simulink model "CSI_0313_4DC"  (R2018a)
settings: Solver=FixedStepDiscrete  StartTime=0.0  StopTime=Tstop  FixedStep=Tdelt  MaxStep=1e-4  RelTol=1e-3
values from neighbouring files (symbols this model uses):
  C = 12e-6    (= 1.2e-05)    [Inputparameter.m]
  Cdc = 4.76*10^-3    (= 0.00476)    [Inputparameter.m]
  Cemc = 1.5e-6    (= 1.5e-06)    [Inputparameter.m]
  fanalog = 7000    [Run.m]
  fKIUdc = 6    [Run.m]
  fKPUdc = 0.4    [Run.m]
  fTs = Update/18000    (= 0.000111111111111)    [Run.m]
  K120 = 0.0    (= 0)    [Run.m]
  K21 = 0.0    (= 0)    [Run.m]
  K5 = 0.0    (= 0)    [Run.m]
  K7 = 0.0    (= 0)    [Run.m]
  Kipll = 1.0    (= 1)    [Run.m]
  klmt = 0.3    [Run.m]
  Kpll = 20.0    (= 20)    [Run.m]
  Lgrid = 7.717e-4*10    (= 0.007717)    [Run.m]
  Lline = 60e-6    (= 6e-05)    [Inputparameter.m]
  Lpwm = 184.8e-6    (= 0.0001848)    [Inputparameter.m]
  mode = 1    [Run.m]
  Nsw = 18000/fbase    [Run.m]
  Qbpf = 1.0    (= 1)    [Run.m]
  Rc = 10e-3    (= 0.01)    [Inputparameter.m]
  Remc = 1e-3    (= 0.001)    [Inputparameter.m]
  Rgrid = 2*pi*fbase*Lgrid/XR    [Run.m]
  Rline = 4.95e-3    (= 0.00495)    [Inputparameter.m]
  Rpre = 2.2    [Inputparameter.m]
  Rpwm = 6.2e-3    (= 0.0062)    [Inputparameter.m]
  Tdelt = (fTs)/(200*Update)    (= 2.77777777778e-07)    [Run.m]
  Tdt = 1.27e-6    (= 1.27e-06)    [Run.m]
  tstart = 0.2    [Run.m]
  Tvstep = 1.5    [Run.m]
  Update = 2    [Run.m]
  Vbase = 400*sqrt(2/3)    [Inputparameter.m]
undefined symbols (not defined in the file or in its folder): sigbuilder_block
libraries: powerlib x412
(part 2 of 13)

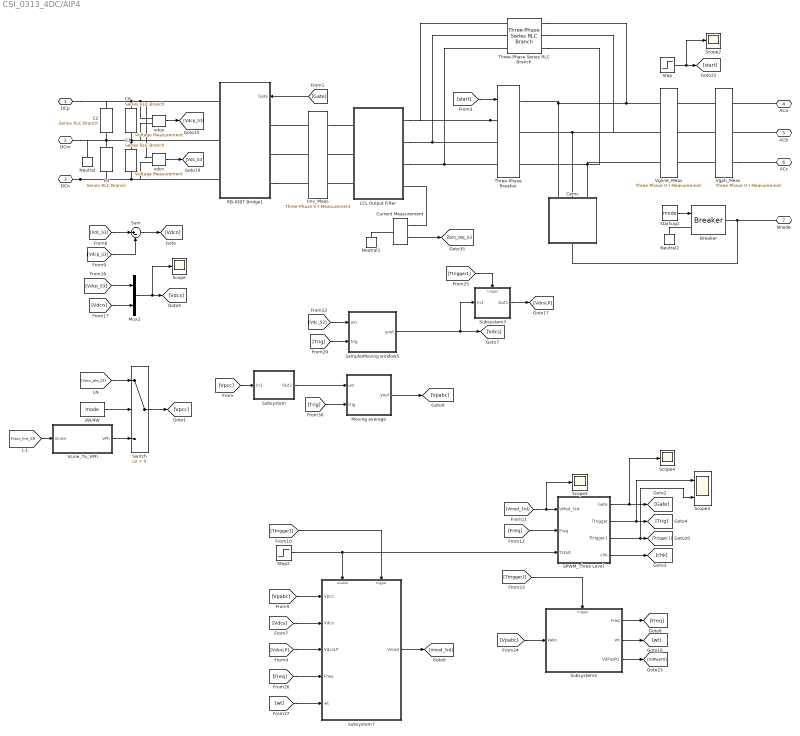
== system CSI_0313_4DC/AIP4 ==
  3W/4W : Constant  Value=mode
  Breaker : powerlib/Elements/Breaker  InitialState=0  SwitchingTimes="[1/60  5/60]"  External=on  BreakerResistance=1e-6  SnubberResistance=1e6  SnubberCapacitance=inf  Measurements=None  MoreParameters=on  NoBreakLoop=off
      settings: SourceProductName=Simscape Electrical
  C1 : powerlib/Elements/Series RLC Branch  LConnTagsString=__new0  RConnTagsString=__new0  BranchType=C  Resistance=Rc  Inductance=Lpwm  SetiL0=off  InitialCurrent=0  Capacitance=Cdc  Setx0=on  InitialVoltage=320  Measurements=None
      settings: SourceProductName=Simscape Electrical
  C2 : powerlib/Elements/Series RLC Branch  LConnTagsString=__new0  RConnTagsString=__new0  BranchType=R  Resistance=120e3  Inductance=Lpwm  SetiL0=off  InitialCurrent=0  Capacitance=Cdc  Setx0=on  InitialVoltage=300  Measurements=None
      settings: SourceProductName=Simscape Electrical
  C3 : powerlib/Elements/Series RLC Branch  LConnTagsString=__new0  RConnTagsString=__new0  BranchType=R  Resistance=120e3  Inductance=Lpwm  SetiL0=off  InitialCurrent=0  Capacitance=Cdc  Setx0=on  InitialVoltage=300  Measurements=None
      settings: SourceProductName=Simscape Electrical
  C8 : powerlib/Elements/Series RLC Branch  LConnTagsString=__new0  RConnTagsString=__new0  BranchType=C  Resistance=Rc  Inductance=Lpwm  SetiL0=off  InitialCurrent=0  Capacitance=Cdc  Setx0=on  InitialVoltage=320  Measurements=None
      settings: SourceProductName=Simscape Electrical
  Cemc : Subsystem
  Current Measurement : powerlib/Measurements/Current Measurement  PhasorSimulation=off  OutputType=Complex  PSBequivalent=0
      settings: SourceProductName=Simscape Electrical
  Iinv_Meas : powerlib/Measurements/Three-Phase V-I Measurement  VoltageMeasurement=no  SetLabelV=off  LabelV=Vabc  Vpu=off  VpuLL=off  CurrentMeasurement=yes  SetLabelI=on  LabelI=Iinv_S3  Ipu=off  Pbase=100e6  Vbase=500e3  OutputType=Complex  PhasorSimulation=off  PSBequivalent=0
      settings: SourceProductName=Simscape Electrical
  LCL Output Filter : Subsystem  AncestorBlock=AIP_Library0107/LCL Output Filter
  Moving average : MATLAB Function  Priority=-1  AncestorBlock=AIP_Library0123/Sample//Moving window  TreatAsAtomicUnit=on  mask{iNumAvg=4, iNumDly=1, ubase=1}
      mask prompts: iNumAvg "Sample points"; iNumDly "Delay points"; ubase "Base Value"
  Mux2 : Mux  Inputs=2
  Neutral : powerlib/Elements/Neutral  LConnTagsString=a  NodeNumber=10
      settings: SourceProductName=Simscape Electrical  SourceProductBaseCode=PS
  Neutral1 : powerlib/Elements/Neutral  LConnTagsString=a  NodeNumber=10
      settings: SourceProductName=Simscape Electrical  SourceProductBaseCode=PS
  Neutral2 : powerlib/Elements/Neutral  LConnTagsString=a  NodeNumber=10
      settings: SourceProductName=Simscape Electrical  SourceProductBaseCode=PS
  RB-IGBT Bridge1 : Subsystem  AncestorBlock=AIP_Library0107/RB-IGBT Bridge
  SPWM_Three Level : Subsystem  mask{ID=1, Tdelt=Tdelt, Tdt=Tdt}
      mask prompts: ID "Unit Serial Number"; Tdelt "Simulation Step [s]"; Tdt "Dead time [s]"
  Sample/Moving window5 : MATLAB Function  Priority=-1  AncestorBlock=AIP_Library0123/Sample//Moving window  TreatAsAtomicUnit=on  mask{iNumAvg=1, iNumDly=1, ubase=1}
      mask prompts: iNumAvg "Sample points"; iNumDly "Delay points"; ubase "Base Value"
  Scope{,2,4..5} (4 alike) : Scope
  Scope3 : Scope  NumInputPorts=2
  Startsig1 : Constant  Value=mode
  Step : Step  Time=0.25  SampleTime=0
  Step2 : Step  Time=0.25  SampleTime=0
  Subsystem : Subsystem
  Subsystem3 : Subsystem
  Subsystem5 : Subsystem
  Subsystem7 : Subsystem
  Sum : Sum  Inputs=|+-
  Switch : Switch  Criteria=u2 > Threshold
  Three-Phase Series RLC Branch : powerlib/Elements/Three-Phase Series RLC Branch  LConnTagsString=A|B|C  RConnTagsString=A|B|C  BranchType=R  Resistance=Rpre  Inductance=1e-3  Capacitance=1e-6  Measurements=None
      settings: SourceProductName=Simscape Electrical
  Three-Phase Breaker : powerlib/Elements/Three-Phase Breaker  InitialState=open  SwitchA=on  SwitchB=on  SwitchC=on  SwitchTimes=tstart  External=on  BreakerResistance=1e-6  SnubberResistance=1e6  SnubberCapacitance=inf  Measurements=None
      settings: SourceProductName=Simscape Electrical
  VLine_To_VPh : MATLAB Function  AncestorBlock=AIP_Library0107/VLine_To_VPh  TreatAsAtomicUnit=on
  Vgline_Meas : powerlib/Measurements/Three-Phase V-I Measurement  VoltageMeasurement=phase-to-phase  SetLabelV=on  LabelV=Vpcc_line_S3  Vpu=off  VpuLL=off  CurrentMeasurement=no  SetLabelI=off  LabelI=vpccabbc  Ipu=off  Pbase=100e6  Vbase=500e3  OutputType=Complex  PhasorSimulation=off  PSBequivalent=0
      settings: SourceProductName=Simscape Electrical
  Vgph_Meas : powerlib/Measurements/Three-Phase V-I Measurement  VoltageMeasurement=phase-to-ground  SetLabelV=on  LabelV=Vpcc_phn_S3  Vpu=off  VpuLL=off  CurrentMeasurement=no  SetLabelI=off  LabelI=vpccabbc  Ipu=off  Pbase=100e6  Vbase=500e3  OutputType=Complex  PhasorSimulation=off  PSBequivalent=0
      settings: SourceProductName=Simscape Electrical
  vdcn : powerlib/Measurements/Voltage Measurement  PhasorSimulation=off  OutputType=Magnitude  PSBequivalent=0
      settings: SourceProductName=Simscape Electrical
  vdcp : powerlib/Measurements/Voltage Measurement  PhasorSimulation=off  OutputType=Magnitude  PSBequivalent=0
      settings: SourceProductName=Simscape Electrical
  DCp : PMIOPort  Side=Left
  DCm : PMIOPort  Port=2  Side=Left
  DCn : PMIOPort  Port=3  Side=Left
  ACa : PMIOPort  Port=4  Side=Right
  ACb : PMIOPort  Port=5  Side=Right
  ACc : PMIOPort  Port=6  Side=Right
  Nnode : PMIOPort  Port=7  Side=Right
  tag scope: Zero_seq_S3=global
  wires:
  [wt] -> Subsystem7/5(wt)
  Subsystem5/3(VdPosPU) -> [VdPosPU]
  Subsystem5/2(wt) -> [wt]
  [Freq] -> Subsystem7/4("Freq ")
  [Vpabc] -> Subsystem5/1(Vabc)
  [Ttrigger1] -> Subsystem5/Trigger
  Sample/Moving window5/1(yout) -> [Vdcs], Subsystem3/1(In1)
  [Vdc_S3] -> Sample/Moving window5/1(uin)
  Sum/1 -> [Vdcn]
  [Vdcp_S3] -> Sum/2
  [Vdc_S3] -> Sum/1
  [VdcsLP] -> Subsystem7/3(VdcsLP)
  Subsystem3/1(Out1) -> [VdcsLP]
  Step2/1 -> Subsystem7/Enable, SPWM_Three Level/3(Tstart)
  [start] -> Three-Phase Breaker/1
  [Ttrigger1] -> Subsystem3/Trigger
  [Trig] -> Sample/Moving window5/2(trig)
  vdcp/1 -> [Vdcp_S3]
  Startsig1/1 -> Breaker/1
  Step/1 -> [start], Scope2/1
  [Gate] -> RB-IGBT Bridge1/1(Gate)
  vdcn/1 -> [Vdc_S3]
  Current Measurement/1 -> [Zero_seq_S3]
  [Freq] -> SPWM_Three Level/2(Freq)
  [Vmod_3rd] -> Scope5/1, SPWM_Three Level/1(VMod_3rd)
  Subsystem5/1(Freq) -> [Freq]
  Subsystem7/1(Vmod) -> [Vmod_3rd]
  [Ttrigger1] -> Subsystem7/Trigger
  [Vdcs] -> Subsystem7/2(Vdcs)
  [Vpabc] -> Subsystem7/1(Vpcc)
  [Vdcn] -> Mux2/2
  [Vdcp_S3] -> Mux2/1
  SPWM_Three Level/4(chk) -> [chk]
  SPWM_Three Level/3(Ttrigger1) -> [Ttrigger1], Scope3/2
  SPWM_Three Level/1(Gate) -> [Gate], Scope4/1
  Mux2/1 -> [Vdcx], Scope/1
  SPWM_Three Level/2(Ttrigger) -> [Trig], Scope3/1
  Switch/1 -> [Vpcc]
  [Vpcc_phn_S3] -> Switch/1
  Subsystem/1(Out1) -> Moving average/1(uin)
  [Trig] -> Moving average/2(trig)
  Moving average/1(yout) -> [Vpabc]
  VLine_To_VPh/1(VPh) -> Switch/3
  [Vpcc_line_S3] -> VLine_To_VPh/1(VLine)
  [Vpcc] -> Subsystem/1(In1)
  3W/4W/1 -> Switch/2
  connections:
  Current Measurement/RConn1 -- LCL Output Filter/RConn4
  LCL Output Filter/LConn3 -- Iinv_Meas/RConn3
  Vgph_Meas/LConn3 -- Vgline_Meas/RConn3
  Vgph_Meas/LConn1 -- Vgline_Meas/RConn1
  LCL Output Filter/LConn2 -- Iinv_Meas/RConn2
  Iinv_Meas/RConn1 -- LCL Output Filter/LConn1
  RB-IGBT Bridge1/LConn1 -- Iinv_Meas/LConn1
  ACb/RConn1 -- Vgph_Meas/RConn2
  Vgph_Meas/LConn2 -- Vgline_Meas/RConn2
  Vgph_Meas/RConn3 -- ACc/RConn1
  RB-IGBT Bridge1/LConn3 -- Iinv_Meas/LConn3
  Neutral2/LConn1 -- Breaker/LConn1
  RB-IGBT Bridge1/LConn2 -- Iinv_Meas/LConn2
  ACa/RConn1 -- Vgph_Meas/RConn1
  Current Measurement/LConn1 -- Neutral1/LConn1
  Three-Phase Breaker/LConn1 -- LCL Output Filter/RConn1 -- Three-Phase Series RLC Branch/LConn1
  DCn/RConn1 -- C3/RConn1 -- C1/RConn1 -- vdcn/LConn2 -- RB-IGBT Bridge1/RConn3
  Nnode/RConn1 -- Breaker/RConn1 -- Cemc/RConn1
  Three-Phase Series RLC Branch/LConn2 -- LCL Output Filter/RConn2 -- Three-Phase Breaker/LConn2
  Cemc/LConn2 -- Three-Phase Series RLC Branch/RConn2 -- Vgline_Meas/LConn2 -- Three-Phase Breaker/RConn2
  Three-Phase Series RLC Branch/LConn3 -- LCL Output Filter/RConn3 -- Three-Phase Breaker/LConn3
  C1/LConn1 -- vdcp/LConn2 -- RB-IGBT Bridge1/RConn2 -- C2/RConn1 -- Neutral/LConn1 -- DCm/RConn1 -- C3/LConn1 -- C8/RConn1
  Cemc/LConn3 -- Three-Phase Series RLC Branch/RConn3 -- Vgline_Meas/LConn3 -- Three-Phase Breaker/RConn3
  Cemc/LConn1 -- Three-Phase Breaker/RConn1 -- Three-Phase Series RLC Branch/RConn1 -- Vgline_Meas/LConn1
  C8/LConn1 -- DCp/RConn1 -- C2/LConn1 -- RB-IGBT Bridge1/RConn1 -- vdcn/LConn1 -- vdcp/LConn1

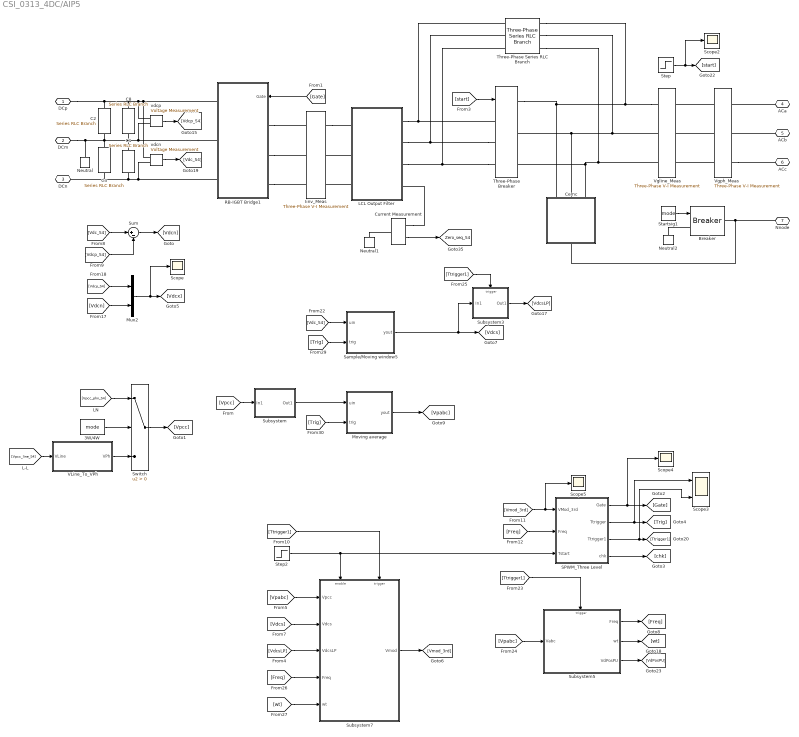
== system CSI_0313_4DC/AIP5 ==
  3W/4W : Constant  Value=mode
  Breaker : powerlib/Elements/Breaker  InitialState=0  SwitchingTimes="[1/60  5/60]"  External=on  BreakerResistance=1e-6  SnubberResistance=1e6  SnubberCapacitance=inf  Measurements=None  MoreParameters=on  NoBreakLoop=off
      settings: SourceProductName=Simscape Electrical
  C1 : powerlib/Elements/Series RLC Branch  LConnTagsString=__new0  RConnTagsString=__new0  BranchType=C  Resistance=Rc  Inductance=Lpwm  SetiL0=off  InitialCurrent=0  Capacitance=Cdc  Setx0=on  InitialVoltage=320  Measurements=None
      settings: SourceProductName=Simscape Electrical
  C2 : powerlib/Elements/Series RLC Branch  LConnTagsString=__new0  RConnTagsString=__new0  BranchType=R  Resistance=120e3  Inductance=Lpwm  SetiL0=off  InitialCurrent=0  Capacitance=Cdc  Setx0=on  InitialVoltage=300  Measurements=None
      settings: SourceProductName=Simscape Electrical
  C3 : powerlib/Elements/Series RLC Branch  LConnTagsString=__new0  RConnTagsString=__new0  BranchType=R  Resistance=120e3  Inductance=Lpwm  SetiL0=off  InitialCurrent=0  Capacitance=Cdc  Setx0=on  InitialVoltage=300  Measurements=None
      settings: SourceProductName=Simscape Electrical
  C8 : powerlib/Elements/Series RLC Branch  LConnTagsString=__new0  RConnTagsString=__new0  BranchType=C  Resistance=Rc  Inductance=Lpwm  SetiL0=off  InitialCurrent=0  Capacitance=Cdc  Setx0=on  InitialVoltage=320  Measurements=None
      settings: SourceProductName=Simscape Electrical
  Cemc : Subsystem
  Current Measurement : powerlib/Measurements/Current Measurement  PhasorSimulation=off  OutputType=Complex  PSBequivalent=0
      settings: SourceProductName=Simscape Electrical
  Iinv_Meas : powerlib/Measurements/Three-Phase V-I Measurement  VoltageMeasurement=no  SetLabelV=off  LabelV=Vabc  Vpu=off  VpuLL=off  CurrentMeasurement=yes  SetLabelI=on  LabelI=Iinv_S4  Ipu=off  Pbase=100e6  Vbase=500e3  OutputType=Complex  PhasorSimulation=off  PSBequivalent=0
      settings: SourceProductName=Simscape Electrical
  LCL Output Filter : Subsystem  AncestorBlock=AIP_Library0107/LCL Output Filter
  Moving average : MATLAB Function  Priority=-1  AncestorBlock=AIP_Library0123/Sample//Moving window  TreatAsAtomicUnit=on  mask{iNumAvg=4, iNumDly=1, ubase=1}
      mask prompts: iNumAvg "Sample points"; iNumDly "Delay points"; ubase "Base Value"
  Mux2 : Mux  Inputs=2
  Neutral : powerlib/Elements/Neutral  LConnTagsString=a  NodeNumber=10
      settings: SourceProductName=Simscape Electrical  SourceProductBaseCode=PS
  Neutral1 : powerlib/Elements/Neutral  LConnTagsString=a  NodeNumber=10
      settings: SourceProductName=Simscape Electrical  SourceProductBaseCode=PS
  Neutral2 : powerlib/Elements/Neutral  LConnTagsString=a  NodeNumber=10
      settings: SourceProductName=Simscape Electrical  SourceProductBaseCode=PS
  RB-IGBT Bridge1 : Subsystem  AncestorBlock=AIP_Library0107/RB-IGBT Bridge
  SPWM_Three Level : Subsystem  mask{ID=1, Tdelt=Tdelt, Tdt=Tdt}
      mask prompts: ID "Unit Serial Number"; Tdelt "Simulation Step [s]"; Tdt "Dead time [s]"
  Sample/Moving window5 : MATLAB Function  Priority=-1  AncestorBlock=AIP_Library0123/Sample//Moving window  TreatAsAtomicUnit=on  mask{iNumAvg=1, iNumDly=1, ubase=1}
      mask prompts: iNumAvg "Sample points"; iNumDly "Delay points"; ubase "Base Value"
  Scope{,2,4..5} (4 alike) : Scope
  Scope3 : Scope  NumInputPorts=2
  Startsig1 : Constant  Value=mode
  Step : Step  Time=0.3  SampleTime=0
  Step2 : Step  Time=0.3  SampleTime=0
  Subsystem : Subsystem
  Subsystem3 : Subsystem
  Subsystem5 : Subsystem
  Subsystem7 : Subsystem
  Sum : Sum  Inputs=|+-
  Switch : Switch  Criteria=u2 > Threshold
  Three-Phase Series RLC Branch : powerlib/Elements/Three-Phase Series RLC Branch  LConnTagsString=A|B|C  RConnTagsString=A|B|C  BranchType=R  Resistance=Rpre  Inductance=1e-3  Capacitance=1e-6  Measurements=None
      settings: SourceProductName=Simscape Electrical
  Three-Phase Breaker : powerlib/Elements/Three-Phase Breaker  InitialState=open  SwitchA=on  SwitchB=on  SwitchC=on  SwitchTimes=tstart  External=on  BreakerResistance=1e-6  SnubberResistance=1e6  SnubberCapacitance=inf  Measurements=None
      settings: SourceProductName=Simscape Electrical
  VLine_To_VPh : MATLAB Function  AncestorBlock=AIP_Library0107/VLine_To_VPh  TreatAsAtomicUnit=on
  Vgline_Meas : powerlib/Measurements/Three-Phase V-I Measurement  VoltageMeasurement=phase-to-phase  SetLabelV=on  LabelV=Vpcc_line_S4  Vpu=off  VpuLL=off  CurrentMeasurement=no  SetLabelI=off  LabelI=vpccabbc  Ipu=off  Pbase=100e6  Vbase=500e3  OutputType=Complex  PhasorSimulation=off  PSBequivalent=0
      settings: SourceProductName=Simscape Electrical
  Vgph_Meas : powerlib/Measurements/Three-Phase V-I Measurement  VoltageMeasurement=phase-to-ground  SetLabelV=on  LabelV=Vpcc_phn_S4  Vpu=off  VpuLL=off  CurrentMeasurement=no  SetLabelI=off  LabelI=vpccabbc  Ipu=off  Pbase=100e6  Vbase=500e3  OutputType=Complex  PhasorSimulation=off  PSBequivalent=0
      settings: SourceProductName=Simscape Electrical
  vdcn : powerlib/Measurements/Voltage Measurement  PhasorSimulation=off  OutputType=Magnitude  PSBequivalent=0
      settings: SourceProductName=Simscape Electrical
  vdcp : powerlib/Measurements/Voltage Measurement  PhasorSimulation=off  OutputType=Magnitude  PSBequivalent=0
      settings: SourceProductName=Simscape Electrical
  DCp : PMIOPort  Side=Left
  DCm : PMIOPort  Port=2  Side=Left
  DCn : PMIOPort  Port=3  Side=Left
  ACa : PMIOPort  Port=4  Side=Right
  ACb : PMIOPort  Port=5  Side=Right
  ACc : PMIOPort  Port=6  Side=Right
  Nnode : PMIOPort  Port=7  Side=Right
  tag scope: Zero_seq_S4=global
  wires:
  SPWM_Three Level/2(Ttrigger) -> Scope3/1, [Trig]
  Mux2/1 -> Scope/1, [Vdcx]
  SPWM_Three Level/1(Gate) -> Scope4/1, [Gate]
  SPWM_Three Level/3(Ttrigger1) -> Scope3/2, [Ttrigger1]
  SPWM_Three Level/4(chk) -> [chk]
  [Vdcp_S4] -> Mux2/1
  [Vdcn] -> Mux2/2
  [Vpabc] -> Subsystem7/1(Vpcc)
  [Vdcs] -> Subsystem7/2(Vdcs)
  [Ttrigger1] -> Subsystem7/Trigger
  Subsystem7/1(Vmod) -> [Vmod_3rd]
  Subsystem5/1(Freq) -> [Freq]
  [Vmod_3rd] -> SPWM_Three Level/1(VMod_3rd), Scope5/1
  [Freq] -> SPWM_Three Level/2(Freq)
  Current Measurement/1 -> [Zero_seq_S4]
  vdcn/1 -> [Vdc_S4]
  [Gate] -> RB-IGBT Bridge1/1(Gate)
  Step/1 -> Scope2/1, [start]
  Startsig1/1 -> Breaker/1
  vdcp/1 -> [Vdcp_S4]
  [Trig] -> Sample/Moving window5/2(trig)
  [Ttrigger1] -> Subsystem3/Trigger
  [start] -> Three-Phase Breaker/1
  Step2/1 -> SPWM_Three Level/3(Tstart), Subsystem7/Enable
  Subsystem3/1(Out1) -> [VdcsLP]
  [VdcsLP] -> Subsystem7/3(VdcsLP)
  [Vdc_S4] -> Sum/1
  [Vdcp_S4] -> Sum/2
  Sum/1 -> [Vdcn]
  [Vdc_S4] -> Sample/Moving window5/1(uin)
  Sample/Moving window5/1(yout) -> Subsystem3/1(In1), [Vdcs]
  [Ttrigger1] -> Subsystem5/Trigger
  [Vpabc] -> Subsystem5/1(Vabc)
  [Freq] -> Subsystem7/4("Freq ")
  Subsystem5/2(wt) -> [wt]
  Subsystem5/3(VdPosPU) -> [VdPosPU]
  [wt] -> Subsystem7/5(wt)
  3W/4W/1 -> Switch/2
  VLine_To_VPh/1(VPh) -> Switch/3
  Moving average/1(yout) -> [Vpabc]
  [Vpcc_phn_S4] -> Switch/1
  [Vpcc] -> Subsystem/1(In1)
  [Trig] -> Moving average/2(trig)
  Subsystem/1(Out1) -> Moving average/1(uin)
  Switch/1 -> [Vpcc]
  [Vpcc_line_S4] -> VLine_To_VPh/1(VLine)
  connections:
  vdcp/LConn1 -- vdcn/LConn1 -- RB-IGBT Bridge1/RConn1 -- C2/LConn1 -- DCp/RConn1 -- C8/LConn1
  Vgline_Meas/LConn1 -- Three-Phase Series RLC Branch/RConn1 -- Three-Phase Breaker/RConn1 -- Cemc/LConn1
  Three-Phase Breaker/RConn3 -- Vgline_Meas/LConn3 -- Three-Phase Series RLC Branch/RConn3 -- Cemc/LConn3
  C8/RConn1 -- C3/LConn1 -- DCm/RConn1 -- Neutral/LConn1 -- C2/RConn1 -- RB-IGBT Bridge1/RConn2 -- vdcp/LConn2 -- C1/LConn1
  Three-Phase Breaker/LConn3 -- LCL Output Filter/RConn3 -- Three-Phase Series RLC Branch/LConn3
  Three-Phase Breaker/RConn2 -- Vgline_Meas/LConn2 -- Three-Phase Series RLC Branch/RConn2 -- Cemc/LConn2
  Three-Phase Breaker/LConn2 -- LCL Output Filter/RConn2 -- Three-Phase Series RLC Branch/LConn2
  Cemc/RConn1 -- Breaker/RConn1 -- Nnode/RConn1
  RB-IGBT Bridge1/RConn3 -- vdcn/LConn2 -- C1/RConn1 -- C3/RConn1 -- DCn/RConn1
  Three-Phase Series RLC Branch/LConn1 -- LCL Output Filter/RConn1 -- Three-Phase Breaker/LConn1
  Current Measurement/LConn1 -- Neutral1/LConn1
  ACa/RConn1 -- Vgph_Meas/RConn1
  RB-IGBT Bridge1/LConn2 -- Iinv_Meas/LConn2
  Neutral2/LConn1 -- Breaker/LConn1
  RB-IGBT Bridge1/LConn3 -- Iinv_Meas/LConn3
  Vgph_Meas/RConn3 -- ACc/RConn1
  Vgph_Meas/LConn2 -- Vgline_Meas/RConn2
  ACb/RConn1 -- Vgph_Meas/RConn2
  RB-IGBT Bridge1/LConn1 -- Iinv_Meas/LConn1
  Iinv_Meas/RConn1 -- LCL Output Filter/LConn1
  LCL Output Filter/LConn2 -- Iinv_Meas/RConn2
  Vgph_Meas/LConn1 -- Vgline_Meas/RConn1
  Vgph_Meas/LConn3 -- Vgline_Meas/RConn3
  LCL Output Filter/LConn3 -- Iinv_Meas/RConn3
  Current Measurement/RConn1 -- LCL Output Filter/RConn4

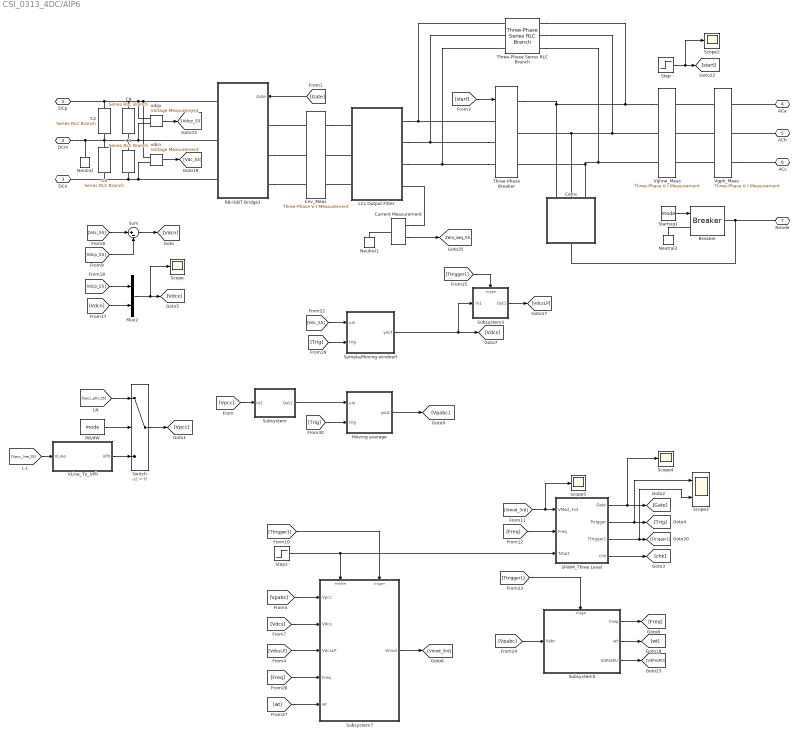
== system CSI_0313_4DC/AIP6 ==
  3W/4W : Constant  Value=mode
  Breaker : powerlib/Elements/Breaker  InitialState=0  SwitchingTimes="[1/60  5/60]"  External=on  BreakerResistance=1e-6  SnubberResistance=1e6  SnubberCapacitance=inf  Measurements=None  MoreParameters=on  NoBreakLoop=off
      settings: SourceProductName=Simscape Electrical
  C1 : powerlib/Elements/Series RLC Branch  LConnTagsString=__new0  RConnTagsString=__new0  BranchType=C  Resistance=Rc  Inductance=Lpwm  SetiL0=off  InitialCurrent=0  Capacitance=Cdc  Setx0=on  InitialVoltage=320  Measurements=None
      settings: SourceProductName=Simscape Electrical
  C2 : powerlib/Elements/Series RLC Branch  LConnTagsString=__new0  RConnTagsString=__new0  BranchType=R  Resistance=120e3  Inductance=Lpwm  SetiL0=off  InitialCurrent=0  Capacitance=Cdc  Setx0=on  InitialVoltage=300  Measurements=None
      settings: SourceProductName=Simscape Electrical
  C3 : powerlib/Elements/Series RLC Branch  LConnTagsString=__new0  RConnTagsString=__new0  BranchType=R  Resistance=120e3  Inductance=Lpwm  SetiL0=off  InitialCurrent=0  Capacitance=Cdc  Setx0=on  InitialVoltage=300  Measurements=None
      settings: SourceProductName=Simscape Electrical
  C8 : powerlib/Elements/Series RLC Branch  LConnTagsString=__new0  RConnTagsString=__new0  BranchType=C  Resistance=Rc  Inductance=Lpwm  SetiL0=off  InitialCurrent=0  Capacitance=Cdc  Setx0=on  InitialVoltage=320  Measurements=None
      settings: SourceProductName=Simscape Electrical
  Cemc : Subsystem
  Current Measurement : powerlib/Measurements/Current Measurement  PhasorSimulation=off  OutputType=Complex  PSBequivalent=0
      settings: SourceProductName=Simscape Electrical
  Iinv_Meas : powerlib/Measurements/Three-Phase V-I Measurement  VoltageMeasurement=no  SetLabelV=off  LabelV=Vabc  Vpu=off  VpuLL=off  CurrentMeasurement=yes  SetLabelI=on  LabelI=Iinv_S5  Ipu=off  Pbase=100e6  Vbase=500e3  OutputType=Complex  PhasorSimulation=off  PSBequivalent=0
      settings: SourceProductName=Simscape Electrical
  LCL Output Filter : Subsystem  AncestorBlock=AIP_Library0107/LCL Output Filter
  Moving average : MATLAB Function  Priority=-1  AncestorBlock=AIP_Library0123/Sample//Moving window  TreatAsAtomicUnit=on  mask{iNumAvg=4, iNumDly=1, ubase=1}
      mask prompts: iNumAvg "Sample points"; iNumDly "Delay points"; ubase "Base Value"
  Mux2 : Mux  Inputs=2
  Neutral : powerlib/Elements/Neutral  LConnTagsString=a  NodeNumber=10
      settings: SourceProductName=Simscape Electrical  SourceProductBaseCode=PS
  Neutral1 : powerlib/Elements/Neutral  LConnTagsString=a  NodeNumber=10
      settings: SourceProductName=Simscape Electrical  SourceProductBaseCode=PS
  Neutral2 : powerlib/Elements/Neutral  LConnTagsString=a  NodeNumber=10
      settings: SourceProductName=Simscape Electrical  SourceProductBaseCode=PS
  RB-IGBT Bridge1 : Subsystem  AncestorBlock=AIP_Library0107/RB-IGBT Bridge
  SPWM_Three Level : Subsystem  mask{ID=1, Tdelt=Tdelt, Tdt=Tdt}
      mask prompts: ID "Unit Serial Number"; Tdelt "Simulation Step [s]"; Tdt "Dead time [s]"
  Sample/Moving window5 : MATLAB Function  Priority=-1  AncestorBlock=AIP_Library0123/Sample//Moving window  TreatAsAtomicUnit=on  mask{iNumAvg=1, iNumDly=1, ubase=1}
      mask prompts: iNumAvg "Sample points"; iNumDly "Delay points"; ubase "Base Value"
  Scope{,2,4..5} (4 alike) : Scope
  Scope3 : Scope  NumInputPorts=2
  Startsig1 : Constant  Value=mode
  Step : Step  Time=0.35  SampleTime=0
  Step2 : Step  Time=0.35  SampleTime=0
  Subsystem : Subsystem
  Subsystem3 : Subsystem
  Subsystem5 : Subsystem
  Subsystem7 : Subsystem
  Sum : Sum  Inputs=|+-
  Switch : Switch  Criteria=u2 > Threshold
  Three-Phase Series RLC Branch : powerlib/Elements/Three-Phase Series RLC Branch  LConnTagsString=A|B|C  RConnTagsString=A|B|C  BranchType=R  Resistance=Rpre  Inductance=1e-3  Capacitance=1e-6  Measurements=None
      settings: SourceProductName=Simscape Electrical
  Three-Phase Breaker : powerlib/Elements/Three-Phase Breaker  InitialState=open  SwitchA=on  SwitchB=on  SwitchC=on  SwitchTimes=tstart  External=on  BreakerResistance=1e-6  SnubberResistance=1e6  SnubberCapacitance=inf  Measurements=None
      settings: SourceProductName=Simscape Electrical
  VLine_To_VPh : MATLAB Function  AncestorBlock=AIP_Library0107/VLine_To_VPh  TreatAsAtomicUnit=on
  Vgline_Meas : powerlib/Measurements/Three-Phase V-I Measurement  VoltageMeasurement=phase-to-phase  SetLabelV=on  LabelV=Vpcc_line_S5  Vpu=off  VpuLL=off  CurrentMeasurement=no  SetLabelI=off  LabelI=vpccabbc  Ipu=off  Pbase=100e6  Vbase=500e3  OutputType=Complex  PhasorSimulation=off  PSBequivalent=0
      settings: SourceProductName=Simscape Electrical
  Vgph_Meas : powerlib/Measurements/Three-Phase V-I Measurement  VoltageMeasurement=phase-to-ground  SetLabelV=on  LabelV=Vpcc_phn_S5  Vpu=off  VpuLL=off  CurrentMeasurement=no  SetLabelI=off  LabelI=vpccabbc  Ipu=off  Pbase=100e6  Vbase=500e3  OutputType=Complex  PhasorSimulation=off  PSBequivalent=0
      settings: SourceProductName=Simscape Electrical
  vdcn : powerlib/Measurements/Voltage Measurement  PhasorSimulation=off  OutputType=Magnitude  PSBequivalent=0
      settings: SourceProductName=Simscape Electrical
  vdcp : powerlib/Measurements/Voltage Measurement  PhasorSimulation=off  OutputType=Magnitude  PSBequivalent=0
      settings: SourceProductName=Simscape Electrical
  DCp : PMIOPort  Side=Left
  DCm : PMIOPort  Port=2  Side=Left
  DCn : PMIOPort  Port=3  Side=Left
  ACa : PMIOPort  Port=4  Side=Right
  ACb : PMIOPort  Port=5  Side=Right
  ACc : PMIOPort  Port=6  Side=Right
  Nnode : PMIOPort  Port=7  Side=Right
  tag scope: Zero_seq_S5=global
  wires:
  SPWM_Three Level/2(Ttrigger) -> Scope3/1, [Trig]
  Mux2/1 -> Scope/1, [Vdcx]
  SPWM_Three Level/1(Gate) -> Scope4/1, [Gate]
  SPWM_Three Level/3(Ttrigger1) -> Scope3/2, [Ttrigger1]
  SPWM_Three Level/4(chk) -> [chk]
  [Vdcp_S5] -> Mux2/1
  [Vdcn] -> Mux2/2
  [Vpabc] -> Subsystem7/1(Vpcc)
  [Vdcs] -> Subsystem7/2(Vdcs)
  [Ttrigger1] -> Subsystem7/Trigger
  Subsystem7/1(Vmod) -> [Vmod_3rd]
  Subsystem5/1(Freq) -> [Freq]
  [Vmod_3rd] -> SPWM_Three Level/1(VMod_3rd), Scope5/1
  [Freq] -> SPWM_Three Level/2(Freq)
  Current Measurement/1 -> [Zero_seq_S5]
  vdcn/1 -> [Vdc_S5]
  [Gate] -> RB-IGBT Bridge1/1(Gate)
  Step/1 -> Scope2/1, [start]
  Startsig1/1 -> Breaker/1
  vdcp/1 -> [Vdcp_S5]
  [Trig] -> Sample/Moving window5/2(trig)
  [Ttrigger1] -> Subsystem3/Trigger
  [start] -> Three-Phase Breaker/1
  Step2/1 -> SPWM_Three Level/3(Tstart), Subsystem7/Enable
  Subsystem3/1(Out1) -> [VdcsLP]
  [VdcsLP] -> Subsystem7/3(VdcsLP)
  [Vdc_S5] -> Sum/1
  [Vdcp_S5] -> Sum/2
  Sum/1 -> [Vdcn]
  [Vdc_S5] -> Sample/Moving window5/1(uin)
  Sample/Moving window5/1(yout) -> Subsystem3/1(In1), [Vdcs]
  [Ttrigger1] -> Subsystem5/Trigger
  [Vpabc] -> Subsystem5/1(Vabc)
  [Freq] -> Subsystem7/4("Freq ")
  Subsystem5/2(wt) -> [wt]
  Subsystem5/3(VdPosPU) -> [VdPosPU]
  [wt] -> Subsystem7/5(wt)
  3W/4W/1 -> Switch/2
  VLine_To_VPh/1(VPh) -> Switch/3
  Moving average/1(yout) -> [Vpabc]
  [Vpcc_phn_S5] -> Switch/1
  [Vpcc] -> Subsystem/1(In1)
  [Trig] -> Moving average/2(trig)
  Subsystem/1(Out1) -> Moving average/1(uin)
  Switch/1 -> [Vpcc]
  [Vpcc_line_S5] -> VLine_To_VPh/1(VLine)
  connections:
  vdcp/LConn1 -- vdcn/LConn1 -- RB-IGBT Bridge1/RConn1 -- C2/LConn1 -- DCp/RConn1 -- C8/LConn1
  Vgline_Meas/LConn1 -- Three-Phase Series RLC Branch/RConn1 -- Three-Phase Breaker/RConn1 -- Cemc/LConn1
  Three-Phase Breaker/RConn3 -- Vgline_Meas/LConn3 -- Three-Phase Series RLC Branch/RConn3 -- Cemc/LConn3
  C8/RConn1 -- C3/LConn1 -- DCm/RConn1 -- Neutral/LConn1 -- C2/RConn1 -- RB-IGBT Bridge1/RConn2 -- vdcp/LConn2 -- C1/LConn1
  Three-Phase Breaker/LConn3 -- LCL Output Filter/RConn3 -- Three-Phase Series RLC Branch/LConn3
  Three-Phase Breaker/RConn2 -- Vgline_Meas/LConn2 -- Three-Phase Series RLC Branch/RConn2 -- Cemc/LConn2
  Three-Phase Breaker/LConn2 -- LCL Output Filter/RConn2 -- Three-Phase Series RLC Branch/LConn2
  Cemc/RConn1 -- Breaker/RConn1 -- Nnode/RConn1
  RB-IGBT Bridge1/RConn3 -- vdcn/LConn2 -- C1/RConn1 -- C3/RConn1 -- DCn/RConn1
  Three-Phase Series RLC Branch/LConn1 -- LCL Output Filter/RConn1 -- Three-Phase Breaker/LConn1
  Current Measurement/LConn1 -- Neutral1/LConn1
  ACa/RConn1 -- Vgph_Meas/RConn1
  RB-IGBT Bridge1/LConn2 -- Iinv_Meas/LConn2
  Neutral2/LConn1 -- Breaker/LConn1
  RB-IGBT Bridge1/LConn3 -- Iinv_Meas/LConn3
  Vgph_Meas/RConn3 -- ACc/RConn1
  Vgph_Meas/LConn2 -- Vgline_Meas/RConn2
  ACb/RConn1 -- Vgph_Meas/RConn2
  RB-IGBT Bridge1/LConn1 -- Iinv_Meas/LConn1
  Iinv_Meas/RConn1 -- LCL Output Filter/LConn1
  LCL Output Filter/LConn2 -- Iinv_Meas/RConn2
  Vgph_Meas/LConn1 -- Vgline_Meas/RConn1
  Vgph_Meas/LConn3 -- Vgline_Meas/RConn3
  LCL Output Filter/LConn3 -- Iinv_Meas/RConn3
  Current Measurement/RConn1 -- LCL Output Filter/RConn4

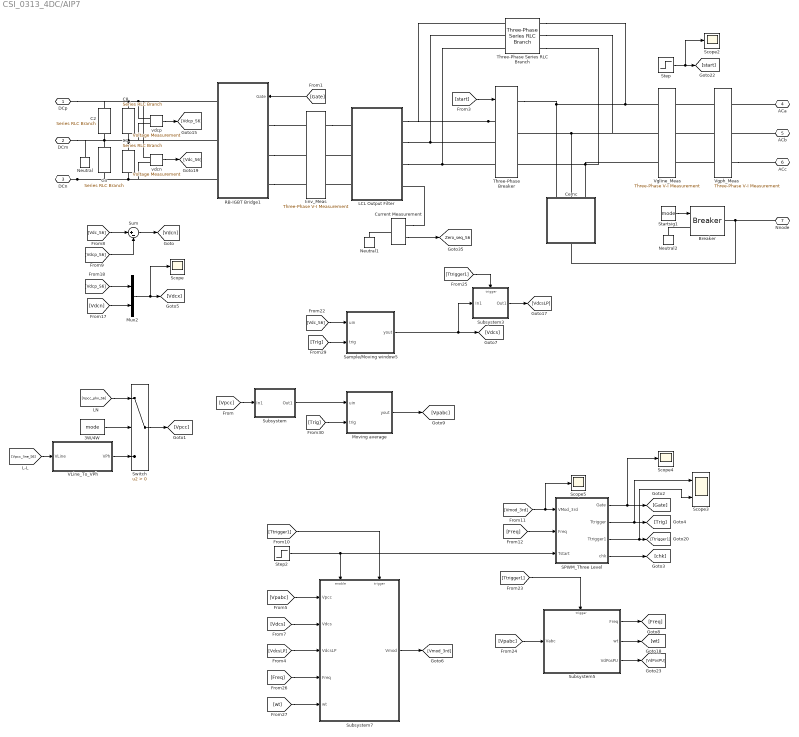
== system CSI_0313_4DC/AIP7 ==
  3W/4W : Constant  Value=mode
  Breaker : powerlib/Elements/Breaker  InitialState=0  SwitchingTimes="[1/60  5/60]"  External=on  BreakerResistance=1e-6  SnubberResistance=1e6  SnubberCapacitance=inf  Measurements=None  MoreParameters=on  NoBreakLoop=off
      settings: SourceProductName=Simscape Electrical
  C1 : powerlib/Elements/Series RLC Branch  LConnTagsString=__new0  RConnTagsString=__new0  BranchType=C  Resistance=Rc  Inductance=Lpwm  SetiL0=off  InitialCurrent=0  Capacitance=Cdc  Setx0=on  InitialVoltage=320  Measurements=None
      settings: SourceProductName=Simscape Electrical
  C2 : powerlib/Elements/Series RLC Branch  LConnTagsString=__new0  RConnTagsString=__new0  BranchType=R  Resistance=120e3  Inductance=Lpwm  SetiL0=off  InitialCurrent=0  Capacitance=Cdc  Setx0=on  InitialVoltage=300  Measurements=None
      settings: SourceProductName=Simscape Electrical
  C3 : powerlib/Elements/Series RLC Branch  LConnTagsString=__new0  RConnTagsString=__new0  BranchType=R  Resistance=120e3  Inductance=Lpwm  SetiL0=off  InitialCurrent=0  Capacitance=Cdc  Setx0=on  InitialVoltage=300  Measurements=None
      settings: SourceProductName=Simscape Electrical
  C8 : powerlib/Elements/Series RLC Branch  LConnTagsString=__new0  RConnTagsString=__new0  BranchType=C  Resistance=Rc  Inductance=Lpwm  SetiL0=off  InitialCurrent=0  Capacitance=Cdc  Setx0=on  InitialVoltage=320  Measurements=None
      settings: SourceProductName=Simscape Electrical
  Cemc : Subsystem
  Current Measurement : powerlib/Measurements/Current Measurement  PhasorSimulation=off  OutputType=Complex  PSBequivalent=0
      settings: SourceProductName=Simscape Electrical
  Iinv_Meas : powerlib/Measurements/Three-Phase V-I Measurement  VoltageMeasurement=no  SetLabelV=off  LabelV=Vabc  Vpu=off  VpuLL=off  CurrentMeasurement=yes  SetLabelI=on  LabelI=Iinv_S6  Ipu=off  Pbase=100e6  Vbase=500e3  OutputType=Complex  PhasorSimulation=off  PSBequivalent=0
      settings: SourceProductName=Simscape Electrical
  LCL Output Filter : Subsystem  AncestorBlock=AIP_Library0107/LCL Output Filter
  Moving average : MATLAB Function  Priority=-1  AncestorBlock=AIP_Library0123/Sample//Moving window  TreatAsAtomicUnit=on  mask{iNumAvg=4, iNumDly=1, ubase=1}
      mask prompts: iNumAvg "Sample points"; iNumDly "Delay points"; ubase "Base Value"
  Mux2 : Mux  Inputs=2
  Neutral : powerlib/Elements/Neutral  LConnTagsString=a  NodeNumber=10
      settings: SourceProductName=Simscape Electrical  SourceProductBaseCode=PS
  Neutral1 : powerlib/Elements/Neutral  LConnTagsString=a  NodeNumber=10
      settings: SourceProductName=Simscape Electrical  SourceProductBaseCode=PS
  Neutral2 : powerlib/Elements/Neutral  LConnTagsString=a  NodeNumber=10
      settings: SourceProductName=Simscape Electrical  SourceProductBaseCode=PS
  RB-IGBT Bridge1 : Subsystem  AncestorBlock=AIP_Library0107/RB-IGBT Bridge
  SPWM_Three Level : Subsystem  mask{ID=1, Tdelt=Tdelt, Tdt=Tdt}
      mask prompts: ID "Unit Serial Number"; Tdelt "Simulation Step [s]"; Tdt "Dead time [s]"
  Sample/Moving window5 : MATLAB Function  Priority=-1  AncestorBlock=AIP_Library0123/Sample//Moving window  TreatAsAtomicUnit=on  mask{iNumAvg=1, iNumDly=1, ubase=1}
      mask prompts: iNumAvg "Sample points"; iNumDly "Delay points"; ubase "Base Value"
  Scope{,2,4..5} (4 alike) : Scope
  Scope3 : Scope  NumInputPorts=2
  Startsig1 : Constant  Value=mode
  Step : Step  Time=0.4  SampleTime=0
  Step2 : Step  Time=0.4  SampleTime=0
  Subsystem : Subsystem
  Subsystem3 : Subsystem
  Subsystem5 : Subsystem
  Subsystem7 : Subsystem
  Sum : Sum  Inputs=|+-
  Switch : Switch  Criteria=u2 > Threshold
  Three-Phase Series RLC Branch : powerlib/Elements/Three-Phase Series RLC Branch  LConnTagsString=A|B|C  RConnTagsString=A|B|C  BranchType=R  Resistance=Rpre  Inductance=1e-3  Capacitance=1e-6  Measurements=None
      settings: SourceProductName=Simscape Electrical
  Three-Phase Breaker : powerlib/Elements/Three-Phase Breaker  InitialState=open  SwitchA=on  SwitchB=on  SwitchC=on  SwitchTimes=tstart  External=on  BreakerResistance=1e-6  SnubberResistance=1e6  SnubberCapacitance=inf  Measurements=None
      settings: SourceProductName=Simscape Electrical
  VLine_To_VPh : MATLAB Function  AncestorBlock=AIP_Library0107/VLine_To_VPh  TreatAsAtomicUnit=on
  Vgline_Meas : powerlib/Measurements/Three-Phase V-I Measurement  VoltageMeasurement=phase-to-phase  SetLabelV=on  LabelV=Vpcc_line_S6  Vpu=off  VpuLL=off  CurrentMeasurement=no  SetLabelI=off  LabelI=vpccabbc  Ipu=off  Pbase=100e6  Vbase=500e3  OutputType=Complex  PhasorSimulation=off  PSBequivalent=0
      settings: SourceProductName=Simscape Electrical
  Vgph_Meas : powerlib/Measurements/Three-Phase V-I Measurement  VoltageMeasurement=phase-to-ground  SetLabelV=on  LabelV=Vpcc_phn_S6  Vpu=off  VpuLL=off  CurrentMeasurement=no  SetLabelI=off  LabelI=vpccabbc  Ipu=off  Pbase=100e6  Vbase=500e3  OutputType=Complex  PhasorSimulation=off  PSBequivalent=0
      settings: SourceProductName=Simscape Electrical
  vdcn : powerlib/Measurements/Voltage Measurement  PhasorSimulation=off  OutputType=Magnitude  PSBequivalent=0
      settings: SourceProductName=Simscape Electrical
  vdcp : powerlib/Measurements/Voltage Measurement  PhasorSimulation=off  OutputType=Magnitude  PSBequivalent=0
      settings: SourceProductName=Simscape Electrical
  DCp : PMIOPort  Side=Left
  DCm : PMIOPort  Port=2  Side=Left
  DCn : PMIOPort  Port=3  Side=Left
  ACa : PMIOPort  Port=4  Side=Right
  ACb : PMIOPort  Port=5  Side=Right
  ACc : PMIOPort  Port=6  Side=Right
  Nnode : PMIOPort  Port=7  Side=Right
  tag scope: Zero_seq_S6=global
  wires:
  [Vpcc_line_S6] -> VLine_To_VPh/1(VLine)
  Switch/1 -> [Vpcc]
  Subsystem/1(Out1) -> Moving average/1(uin)
  [Trig] -> Moving average/2(trig)
  [Vpcc] -> Subsystem/1(In1)
  [Vpcc_phn_S6] -> Switch/1
  Moving average/1(yout) -> [Vpabc]
  VLine_To_VPh/1(VPh) -> Switch/3
  3W/4W/1 -> Switch/2
  [wt] -> Subsystem7/5(wt)
  Subsystem5/3(VdPosPU) -> [VdPosPU]
  Subsystem5/2(wt) -> [wt]
  [Freq] -> Subsystem7/4("Freq ")
  [Vpabc] -> Subsystem5/1(Vabc)
  [Ttrigger1] -> Subsystem5/Trigger
  Sample/Moving window5/1(yout) -> [Vdcs], Subsystem3/1(In1)
  [Vdc_S6] -> Sample/Moving window5/1(uin)
  Sum/1 -> [Vdcn]
  [Vdcp_S6] -> Sum/2
  [Vdc_S6] -> Sum/1
  [VdcsLP] -> Subsystem7/3(VdcsLP)
  Subsystem3/1(Out1) -> [VdcsLP]
  Step2/1 -> Subsystem7/Enable, SPWM_Three Level/3(Tstart)
  [start] -> Three-Phase Breaker/1
  [Ttrigger1] -> Subsystem3/Trigger
  [Trig] -> Sample/Moving window5/2(trig)
  vdcp/1 -> [Vdcp_S6]
  Startsig1/1 -> Breaker/1
  Step/1 -> [start], Scope2/1
  [Gate] -> RB-IGBT Bridge1/1(Gate)
  vdcn/1 -> [Vdc_S6]
  Current Measurement/1 -> [Zero_seq_S6]
  [Freq] -> SPWM_Three Level/2(Freq)
  [Vmod_3rd] -> Scope5/1, SPWM_Three Level/1(VMod_3rd)
  Subsystem5/1(Freq) -> [Freq]
  Subsystem7/1(Vmod) -> [Vmod_3rd]
  [Ttrigger1] -> Subsystem7/Trigger
  [Vdcs] -> Subsystem7/2(Vdcs)
  [Vpabc] -> Subsystem7/1(Vpcc)
  [Vdcn] -> Mux2/2
  [Vdcp_S6] -> Mux2/1
  SPWM_Three Level/4(chk) -> [chk]
  SPWM_Three Level/3(Ttrigger1) -> [Ttrigger1], Scope3/2
  SPWM_Three Level/1(Gate) -> [Gate], Scope4/1
  Mux2/1 -> [Vdcx], Scope/1
  SPWM_Three Level/2(Ttrigger) -> [Trig], Scope3/1
  connections:
  Current Measurement/RConn1 -- LCL Output Filter/RConn4
  LCL Output Filter/LConn3 -- Iinv_Meas/RConn3
  Vgph_Meas/LConn3 -- Vgline_Meas/RConn3
  Vgph_Meas/LConn1 -- Vgline_Meas/RConn1
  LCL Output Filter/LConn2 -- Iinv_Meas/RConn2
  Iinv_Meas/RConn1 -- LCL Output Filter/LConn1
  RB-IGBT Bridge1/LConn1 -- Iinv_Meas/LConn1
  ACb/RConn1 -- Vgph_Meas/RConn2
  Vgph_Meas/LConn2 -- Vgline_Meas/RConn2
  Vgph_Meas/RConn3 -- ACc/RConn1
  RB-IGBT Bridge1/LConn3 -- Iinv_Meas/LConn3
  Neutral2/LConn1 -- Breaker/LConn1
  RB-IGBT Bridge1/LConn2 -- Iinv_Meas/LConn2
  ACa/RConn1 -- Vgph_Meas/RConn1
  Current Measurement/LConn1 -- Neutral1/LConn1
  Three-Phase Breaker/LConn1 -- LCL Output Filter/RConn1 -- Three-Phase Series RLC Branch/LConn1
  DCn/RConn1 -- C3/RConn1 -- C1/RConn1 -- vdcn/LConn2 -- RB-IGBT Bridge1/RConn3
  Nnode/RConn1 -- Breaker/RConn1 -- Cemc/RConn1
  Three-Phase Series RLC Branch/LConn2 -- LCL Output Filter/RConn2 -- Three-Phase Breaker/LConn2
  Cemc/LConn2 -- Three-Phase Series RLC Branch/RConn2 -- Vgline_Meas/LConn2 -- Three-Phase Breaker/RConn2
  Three-Phase Series RLC Branch/LConn3 -- LCL Output Filter/RConn3 -- Three-Phase Breaker/LConn3
  C1/LConn1 -- vdcp/LConn2 -- RB-IGBT Bridge1/RConn2 -- C2/RConn1 -- Neutral/LConn1 -- DCm/RConn1 -- C3/LConn1 -- C8/RConn1
  Cemc/LConn3 -- Three-Phase Series RLC Branch/RConn3 -- Vgline_Meas/LConn3 -- Three-Phase Breaker/RConn3
  Cemc/LConn1 -- Three-Phase Breaker/RConn1 -- Three-Phase Series RLC Branch/RConn1 -- Vgline_Meas/LConn1
  C8/LConn1 -- DCp/RConn1 -- C2/LConn1 -- RB-IGBT Bridge1/RConn1 -- vdcn/LConn1 -- vdcp/LConn1

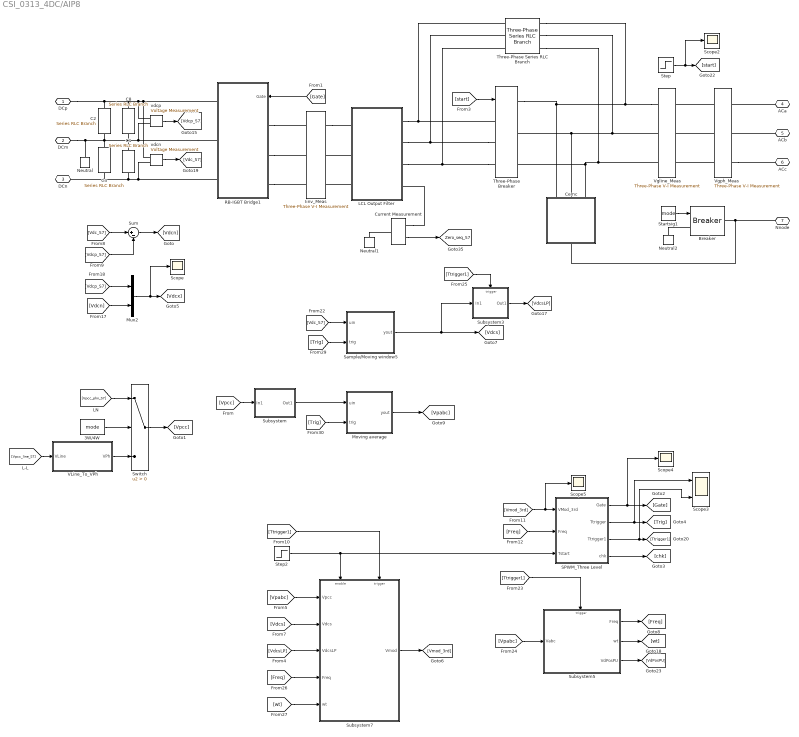
== system CSI_0313_4DC/AIP8 ==
  3W/4W : Constant  Value=mode
  Breaker : powerlib/Elements/Breaker  InitialState=0  SwitchingTimes="[1/60  5/60]"  External=on  BreakerResistance=1e-6  SnubberResistance=1e6  SnubberCapacitance=inf  Measurements=None  MoreParameters=on  NoBreakLoop=off
      settings: SourceProductName=Simscape Electrical
  C1 : powerlib/Elements/Series RLC Branch  LConnTagsString=__new0  RConnTagsString=__new0  BranchType=C  Resistance=Rc  Inductance=Lpwm  SetiL0=off  InitialCurrent=0  Capacitance=Cdc  Setx0=on  InitialVoltage=320  Measurements=None
      settings: SourceProductName=Simscape Electrical
  C2 : powerlib/Elements/Series RLC Branch  LConnTagsString=__new0  RConnTagsString=__new0  BranchType=R  Resistance=120e3  Inductance=Lpwm  SetiL0=off  InitialCurrent=0  Capacitance=Cdc  Setx0=on  InitialVoltage=300  Measurements=None
      settings: SourceProductName=Simscape Electrical
  C3 : powerlib/Elements/Series RLC Branch  LConnTagsString=__new0  RConnTagsString=__new0  BranchType=R  Resistance=120e3  Inductance=Lpwm  SetiL0=off  InitialCurrent=0  Capacitance=Cdc  Setx0=on  InitialVoltage=300  Measurements=None
      settings: SourceProductName=Simscape Electrical
  C8 : powerlib/Elements/Series RLC Branch  LConnTagsString=__new0  RConnTagsString=__new0  BranchType=C  Resistance=Rc  Inductance=Lpwm  SetiL0=off  InitialCurrent=0  Capacitance=Cdc  Setx0=on  InitialVoltage=320  Measurements=None
      settings: SourceProductName=Simscape Electrical
  Cemc : Subsystem
  Current Measurement : powerlib/Measurements/Current Measurement  PhasorSimulation=off  OutputType=Complex  PSBequivalent=0
      settings: SourceProductName=Simscape Electrical
  Iinv_Meas : powerlib/Measurements/Three-Phase V-I Measurement  VoltageMeasurement=no  SetLabelV=off  LabelV=Vabc  Vpu=off  VpuLL=off  CurrentMeasurement=yes  SetLabelI=on  LabelI=Iinv_S7  Ipu=off  Pbase=100e6  Vbase=500e3  OutputType=Complex  PhasorSimulation=off  PSBequivalent=0
      settings: SourceProductName=Simscape Electrical
  LCL Output Filter : Subsystem  AncestorBlock=AIP_Library0107/LCL Output Filter
  Moving average : MATLAB Function  Priority=-1  AncestorBlock=AIP_Library0123/Sample//Moving window  TreatAsAtomicUnit=on  mask{iNumAvg=4, iNumDly=1, ubase=1}
      mask prompts: iNumAvg "Sample points"; iNumDly "Delay points"; ubase "Base Value"
  Mux2 : Mux  Inputs=2
  Neutral : powerlib/Elements/Neutral  LConnTagsString=a  NodeNumber=10
      settings: SourceProductName=Simscape Electrical  SourceProductBaseCode=PS
  Neutral1 : powerlib/Elements/Neutral  LConnTagsString=a  NodeNumber=10
      settings: SourceProductName=Simscape Electrical  SourceProductBaseCode=PS
  Neutral2 : powerlib/Elements/Neutral  LConnTagsString=a  NodeNumber=10
      settings: SourceProductName=Simscape Electrical  SourceProductBaseCode=PS
  RB-IGBT Bridge1 : Subsystem  AncestorBlock=AIP_Library0107/RB-IGBT Bridge
  SPWM_Three Level : Subsystem  mask{ID=1, Tdelt=Tdelt, Tdt=Tdt}
      mask prompts: ID "Unit Serial Number"; Tdelt "Simulation Step [s]"; Tdt "Dead time [s]"
  Sample/Moving window5 : MATLAB Function  Priority=-1  AncestorBlock=AIP_Library0123/Sample//Moving window  TreatAsAtomicUnit=on  mask{iNumAvg=1, iNumDly=1, ubase=1}
      mask prompts: iNumAvg "Sample points"; iNumDly "Delay points"; ubase "Base Value"
  Scope{,2,4..5} (4 alike) : Scope
  Scope3 : Scope  NumInputPorts=2
  Startsig1 : Constant  Value=mode
  Step : Step  Time=0.45  SampleTime=0
  Step2 : Step  Time=0.45  SampleTime=0
  Subsystem : Subsystem
  Subsystem3 : Subsystem
  Subsystem5 : Subsystem
  Subsystem7 : Subsystem
  Sum : Sum  Inputs=|+-
  Switch : Switch  Criteria=u2 > Threshold
  Three-Phase Series RLC Branch : powerlib/Elements/Three-Phase Series RLC Branch  LConnTagsString=A|B|C  RConnTagsString=A|B|C  BranchType=R  Resistance=Rpre  Inductance=1e-3  Capacitance=1e-6  Measurements=None
      settings: SourceProductName=Simscape Electrical
  Three-Phase Breaker : powerlib/Elements/Three-Phase Breaker  InitialState=open  SwitchA=on  SwitchB=on  SwitchC=on  SwitchTimes=tstart  External=on  BreakerResistance=1e-6  SnubberResistance=1e6  SnubberCapacitance=inf  Measurements=None
      settings: SourceProductName=Simscape Electrical
  VLine_To_VPh : MATLAB Function  AncestorBlock=AIP_Library0107/VLine_To_VPh  TreatAsAtomicUnit=on
  Vgline_Meas : powerlib/Measurements/Three-Phase V-I Measurement  VoltageMeasurement=phase-to-phase  SetLabelV=on  LabelV=Vpcc_line_S7  Vpu=off  VpuLL=off  CurrentMeasurement=no  SetLabelI=off  LabelI=vpccabbc  Ipu=off  Pbase=100e6  Vbase=500e3  OutputType=Complex  PhasorSimulation=off  PSBequivalent=0
      settings: SourceProductName=Simscape Electrical
  Vgph_Meas : powerlib/Measurements/Three-Phase V-I Measurement  VoltageMeasurement=phase-to-ground  SetLabelV=on  LabelV=Vpcc_phn_S7  Vpu=off  VpuLL=off  CurrentMeasurement=no  SetLabelI=off  LabelI=vpccabbc  Ipu=off  Pbase=100e6  Vbase=500e3  OutputType=Complex  PhasorSimulation=off  PSBequivalent=0
      settings: SourceProductName=Simscape Electrical
  vdcn : powerlib/Measurements/Voltage Measurement  PhasorSimulation=off  OutputType=Magnitude  PSBequivalent=0
      settings: SourceProductName=Simscape Electrical
  vdcp : powerlib/Measurements/Voltage Measurement  PhasorSimulation=off  OutputType=Magnitude  PSBequivalent=0
      settings: SourceProductName=Simscape Electrical
  DCp : PMIOPort  Side=Left
  DCm : PMIOPort  Port=2  Side=Left
  DCn : PMIOPort  Port=3  Side=Left
  ACa : PMIOPort  Port=4  Side=Right
  ACb : PMIOPort  Port=5  Side=Right
  ACc : PMIOPort  Port=6  Side=Right
  Nnode : PMIOPort  Port=7  Side=Right
  tag scope: Zero_seq_S7=global
  wires:
  SPWM_Three Level/2(Ttrigger) -> Scope3/1, [Trig]
  Mux2/1 -> Scope/1, [Vdcx]
  SPWM_Three Level/1(Gate) -> Scope4/1, [Gate]
  SPWM_Three Level/3(Ttrigger1) -> Scope3/2, [Ttrigger1]
  SPWM_Three Level/4(chk) -> [chk]
  [Vdcp_S7] -> Mux2/1
  [Vdcn] -> Mux2/2
  [Vpabc] -> Subsystem7/1(Vpcc)
  [Vdcs] -> Subsystem7/2(Vdcs)
  [Ttrigger1] -> Subsystem7/Trigger
  Subsystem7/1(Vmod) -> [Vmod_3rd]
  Subsystem5/1(Freq) -> [Freq]
  [Vmod_3rd] -> SPWM_Three Level/1(VMod_3rd), Scope5/1
  [Freq] -> SPWM_Three Level/2(Freq)
  Current Measurement/1 -> [Zero_seq_S7]
  vdcn/1 -> [Vdc_S7]
  [Gate] -> RB-IGBT Bridge1/1(Gate)
  Step/1 -> Scope2/1, [start]
  Startsig1/1 -> Breaker/1
  vdcp/1 -> [Vdcp_S7]
  [Trig] -> Sample/Moving window5/2(trig)
  [Ttrigger1] -> Subsystem3/Trigger
  [start] -> Three-Phase Breaker/1
  Step2/1 -> SPWM_Three Level/3(Tstart), Subsystem7/Enable
  Subsystem3/1(Out1) -> [VdcsLP]
  [VdcsLP] -> Subsystem7/3(VdcsLP)
  [Vdc_S7] -> Sum/1
  [Vdcp_S7] -> Sum/2
  Sum/1 -> [Vdcn]
  [Vdc_S7] -> Sample/Moving window5/1(uin)
  Sample/Moving window5/1(yout) -> [Vdcs], Subsystem3/1(In1)
  [Ttrigger1] -> Subsystem5/Trigger
  [Vpabc] -> Subsystem5/1(Vabc)
  [Freq] -> Subsystem7/4("Freq ")
  Subsystem5/2(wt) -> [wt]
  Subsystem5/3(VdPosPU) -> [VdPosPU]
  [wt] -> Subsystem7/5(wt)
  3W/4W/1 -> Switch/2
  VLine_To_VPh/1(VPh) -> Switch/3
  Moving average/1(yout) -> [Vpabc]
  [Vpcc_phn_S7] -> Switch/1
  [Vpcc] -> Subsystem/1(In1)
  [Trig] -> Moving average/2(trig)
  Subsystem/1(Out1) -> Moving average/1(uin)
  Switch/1 -> [Vpcc]
  [Vpcc_line_S7] -> VLine_To_VPh/1(VLine)
  connections:
  vdcp/LConn1 -- vdcn/LConn1 -- RB-IGBT Bridge1/RConn1 -- C2/LConn1 -- DCp/RConn1 -- C8/LConn1
  Vgline_Meas/LConn1 -- Three-Phase Series RLC Branch/RConn1 -- Three-Phase Breaker/RConn1 -- Cemc/LConn1
  Three-Phase Breaker/RConn3 -- Vgline_Meas/LConn3 -- Three-Phase Series RLC Branch/RConn3 -- Cemc/LConn3
  C8/RConn1 -- C3/LConn1 -- DCm/RConn1 -- Neutral/LConn1 -- C2/RConn1 -- RB-IGBT Bridge1/RConn2 -- vdcp/LConn2 -- C1/LConn1
  Three-Phase Breaker/LConn3 -- LCL Output Filter/RConn3 -- Three-Phase Series RLC Branch/LConn3
  Three-Phase Breaker/RConn2 -- Vgline_Meas/LConn2 -- Three-Phase Series RLC Branch/RConn2 -- Cemc/LConn2
  Three-Phase Breaker/LConn2 -- LCL Output Filter/RConn2 -- Three-Phase Series RLC Branch/LConn2
  Cemc/RConn1 -- Breaker/RConn1 -- Nnode/RConn1
  RB-IGBT Bridge1/RConn3 -- vdcn/LConn2 -- C1/RConn1 -- C3/RConn1 -- DCn/RConn1
  Three-Phase Series RLC Branch/LConn1 -- LCL Output Filter/RConn1 -- Three-Phase Breaker/LConn1
  Current Measurement/LConn1 -- Neutral1/LConn1
  ACa/RConn1 -- Vgph_Meas/RConn1
  RB-IGBT Bridge1/LConn2 -- Iinv_Meas/LConn2
  Neutral2/LConn1 -- Breaker/LConn1
  RB-IGBT Bridge1/LConn3 -- Iinv_Meas/LConn3
  Vgph_Meas/RConn3 -- ACc/RConn1
  Vgph_Meas/LConn2 -- Vgline_Meas/RConn2
  ACb/RConn1 -- Vgph_Meas/RConn2
  RB-IGBT Bridge1/LConn1 -- Iinv_Meas/LConn1
  Iinv_Meas/RConn1 -- LCL Output Filter/LConn1
  LCL Output Filter/LConn2 -- Iinv_Meas/RConn2
  Vgph_Meas/LConn1 -- Vgline_Meas/RConn1
  Vgph_Meas/LConn3 -- Vgline_Meas/RConn3
  LCL Output Filter/LConn3 -- Iinv_Meas/RConn3
  Current Measurement/RConn1 -- LCL Output Filter/RConn4
